simulink model "joint_test"  (R2022a)
settings: Solver=FixedStepAuto  StartTime=0.0  StopTime=2  FixedStep=0.001  RelTol=1e-3
undefined symbols (not defined in the file or in its folder): duration, effort, fins_rev1, index, joint_name, model_missile, model_name
libraries: robotlib x21, simulink_extras x8, robotgazebolib x5, simulink x1
settings Model: Creator=abiyyumufti  LastModifiedBy=abiyyumufti

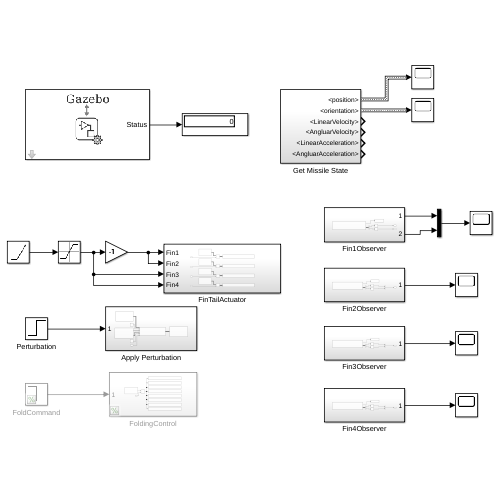
[thumbnail: Simulink's stored preview of the top-level diagram]
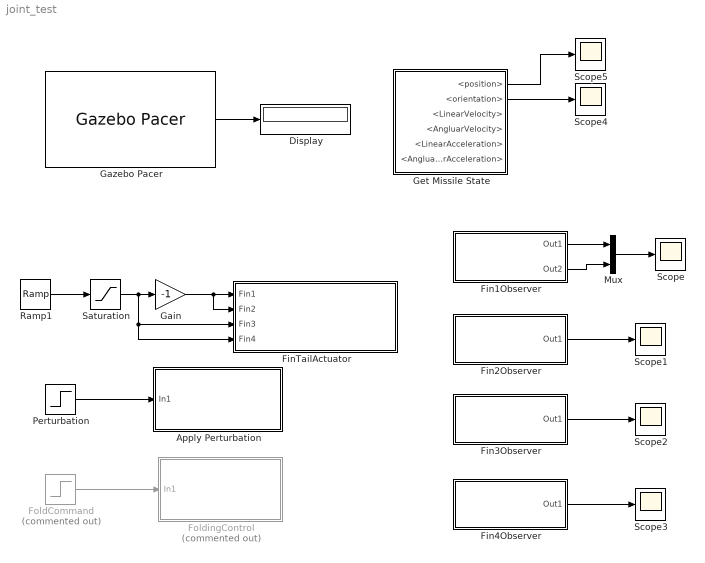
== system joint_test ==
  Apply Perturbation : Subsystem
  Display : Display
  Fin1Observer : Subsystem
  Fin2Observer : Subsystem
  Fin3Observer : Subsystem
  Fin4Observer : Subsystem
  FinTailActuator : Subsystem
  FoldCommand : Step  Commented=on  Time=0.5  Before=deg2rad(123)  After=0  SampleTime=0
  FoldingControl : Subsystem  Commented=on
  Gain : Gain  Gain=-1
  Gazebo Pacer : robotgazebolib/Gazebo Pacer  ResetBehavior=Reset Gazebo simulation time and scene  SampleTime=0.001
      settings: SourceProductBaseCode=RO
  Get Missile State : Subsystem
  Mux : Mux  Inputs=2
  Perturbation : Step  Time=0.25  After=2000  SampleTime=0.001
  Ramp1 : simulink/Sources/Ramp  slope=deg2rad(20)/1  start=0.5  InitialOutput=0
  Saturation : Saturate  UpperLimit=deg2rad(20)  LowerLimit=-deg2rad(20)
  Scope{,1..5} (6 alike) : Scope
  wires:
  Gazebo Pacer/1 -> Display/1
  Perturbation/1 -> Apply Perturbation/1(In1)
  Gain/1 -> FinTailActuator/2(Fin2), FinTailActuator/1(Fin1)
  Saturation/1 -> FinTailActuator/4(Fin4), FinTailActuator/3(Fin3), Gain/1
  Fin4Observer/1(Out1) -> Scope3/1
  Fin3Observer/1(Out1) -> Scope2/1
  Fin2Observer/1(Out1) -> Scope1/1
  Ramp1/1 -> Saturation/1
  FoldCommand/1 -> FoldingControl/1(In1)
  Get Missile State/2(<orientation>) -> Scope4/1
  Get Missile State/1(<position>) -> Scope5/1
  Fin1Observer/1(Out1) -> Mux/1
  Fin1Observer/2(Out2) -> Mux/2
  Mux/1 -> Scope/1

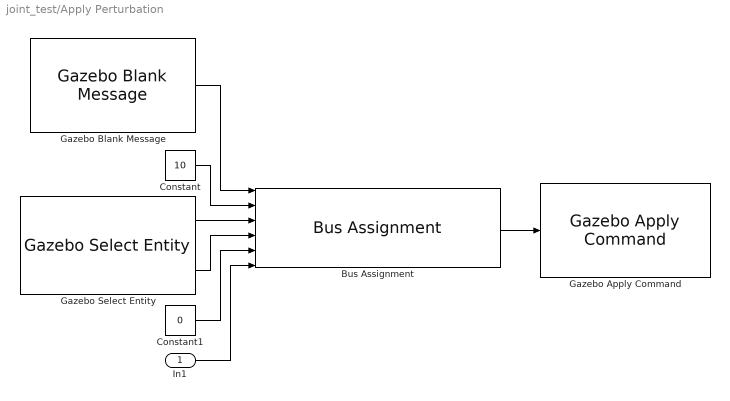
== system joint_test/Apply Perturbation ==
  In1 : Inport
  Bus Assignment : BusAssignment  AssignedSignals=duration.seconds,model_name,joint_name,index,effort
  Constant : Constant  Value=10
  Constant1 : Constant  Value=0  OutDataTypeStr=uint32
  Gazebo Apply Command : robotgazebolib/Gazebo Apply Command  cmdType=ApplyJointTorque  sampleTime=0.001
      settings: SourceProductBaseCode=RO
  Gazebo Blank Message : robotgazebolib/Gazebo Blank Message  msgType=ApplyJointTorque  sampleTime=0.001  busName='Gazebo_SL_Bus_gazebo_msgs_ApplyJointTorque'
      settings: SourceProductBaseCode=RO
  Gazebo Select Entity : robotgazebolib/Gazebo Select Entity  modelElemName=model_missile/fins_rev1  outputArraySize=128  OutputLabel=Joint  SelectType=Joint
      settings: SourceProductBaseCode=RO
  wires:
  Gazebo Select Entity/1 -> Bus Assignment/3
  Constant1/1 -> Bus Assignment/5
  In1/1 -> Bus Assignment/6
  Gazebo Select Entity/2 -> Bus Assignment/4
  Gazebo Blank Message/1 -> Bus Assignment/1
  Bus Assignment/1 -> Gazebo Apply Command/1
  Constant/1 -> Bus Assignment/2

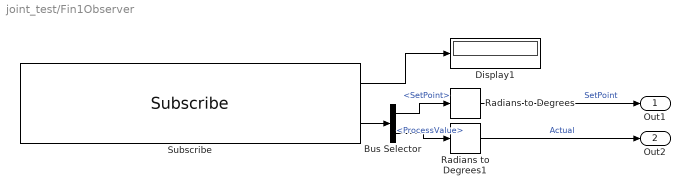
== system joint_test/Fin1Observer ==
  Bus Selector : BusSelector  OutputSignals=SetPoint,ProcessValue
  Display1 : Display
  Radians to Degrees : simulink_extras/Transformations/Radians to Degrees
  Radians to Degrees1 : simulink_extras/Transformations/Radians to Degrees
  Subscribe : robotlib/Subscribe  topicSource=Select from ROS network  topic=/model_missile_controller/fins_rev1_position_controller/state  messageType=control_msgs/JointControllerState  SampleTime=-1  legacyBusStruct=off  messageQueueLength=1
  Out1 : Outport
  Out2 : Outport  Port=2
  wires:
  Subscribe/2 -> Bus Selector/1
  Bus Selector/2 -> Radians to Degrees1/1  "<ProcessValue>"
  Subscribe/1 -> Display1/1
  Bus Selector/1 -> Radians to Degrees/1  "<SetPoint>"
  Radians to Degrees1/1 -> Out2/1  "Actual"
  Radians to Degrees/1 -> Out1/1  "SetPoint"

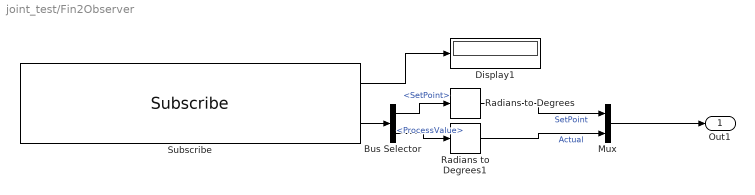
== system joint_test/Fin2Observer ==
  Bus Selector : BusSelector  OutputSignals=SetPoint,ProcessValue
  Display1 : Display
  Mux : Mux  Inputs=2
  Radians to Degrees : simulink_extras/Transformations/Radians to Degrees
  Radians to Degrees1 : simulink_extras/Transformations/Radians to Degrees
  Subscribe : robotlib/Subscribe  topicSource=Select from ROS network  topic=/model_missile_controller/fins_rev2_position_controller/state  messageType=control_msgs/JointControllerState  SampleTime=-1  legacyBusStruct=off  messageQueueLength=1
  Out1 : Outport
  wires:
  Radians to Degrees/1 -> Mux/1  "SetPoint"
  Mux/1 -> Out1/1
  Radians to Degrees1/1 -> Mux/2  "Actual"
  Bus Selector/1 -> Radians to Degrees/1  "<SetPoint>"
  Subscribe/1 -> Display1/1
  Bus Selector/2 -> Radians to Degrees1/1  "<ProcessValue>"
  Subscribe/2 -> Bus Selector/1

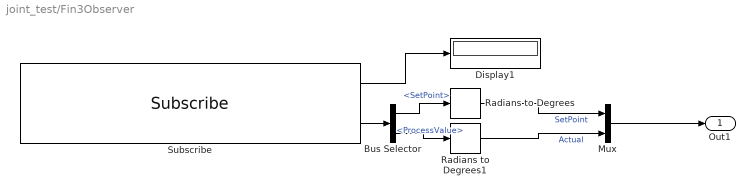
== system joint_test/Fin3Observer ==
  Bus Selector : BusSelector  OutputSignals=SetPoint,ProcessValue
  Display1 : Display
  Mux : Mux  Inputs=2
  Radians to Degrees : simulink_extras/Transformations/Radians to Degrees
  Radians to Degrees1 : simulink_extras/Transformations/Radians to Degrees
  Subscribe : robotlib/Subscribe  topicSource=Select from ROS network  topic=/model_missile_controller/fins_rev3_position_controller/state  messageType=control_msgs/JointControllerState  SampleTime=-1  legacyBusStruct=off  messageQueueLength=1
  Out1 : Outport
  wires:
  Radians to Degrees/1 -> Mux/1  "SetPoint"
  Mux/1 -> Out1/1
  Radians to Degrees1/1 -> Mux/2  "Actual"
  Bus Selector/1 -> Radians to Degrees/1  "<SetPoint>"
  Subscribe/1 -> Display1/1
  Bus Selector/2 -> Radians to Degrees1/1  "<ProcessValue>"
  Subscribe/2 -> Bus Selector/1

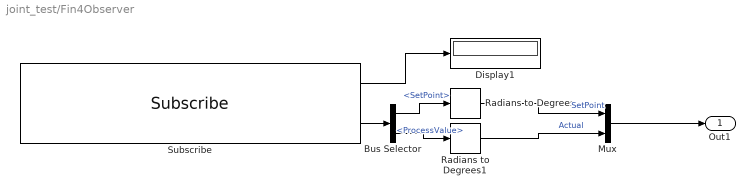
== system joint_test/Fin4Observer ==
  Bus Selector : BusSelector  OutputSignals=SetPoint,ProcessValue
  Display1 : Display
  Mux : Mux  Inputs=2
  Radians to Degrees : simulink_extras/Transformations/Radians to Degrees
  Radians to Degrees1 : simulink_extras/Transformations/Radians to Degrees
  Subscribe : robotlib/Subscribe  topicSource=Select from ROS network  topic=/model_missile_controller/fins_rev4_position_controller/state  messageType=control_msgs/JointControllerState  SampleTime=-1  legacyBusStruct=off  messageQueueLength=1
  Out1 : Outport
  wires:
  Subscribe/2 -> Bus Selector/1
  Bus Selector/2 -> Radians to Degrees1/1  "<ProcessValue>"
  Subscribe/1 -> Display1/1
  Bus Selector/1 -> Radians to Degrees/1  "<SetPoint>"
  Radians to Degrees1/1 -> Mux/2  "Actual"
  Mux/1 -> Out1/1
  Radians to Degrees/1 -> Mux/1  "SetPoint"

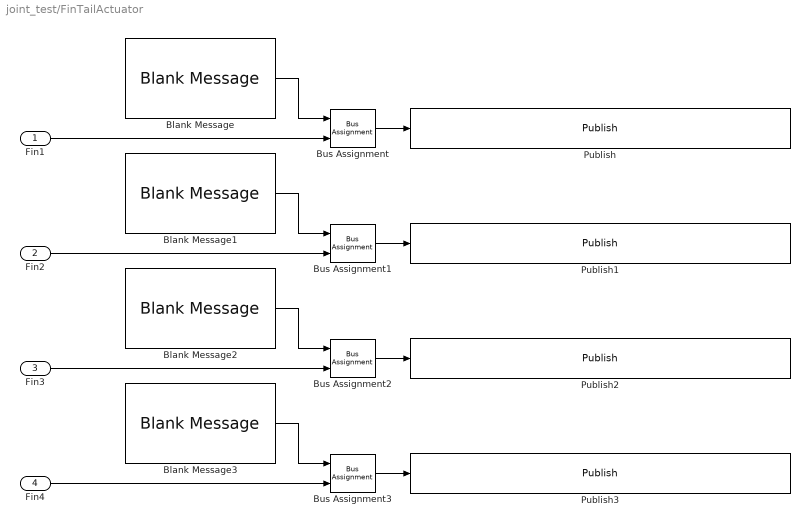
== system joint_test/FinTailActuator ==
  Fin1 : Inport
  Fin2 : Inport  Port=2
  Fin3 : Inport  Port=3
  Fin4 : Inport  Port=4
  Blank Message{,1..3} (4 alike) : robotlib/Blank Message  messageClass=Message  entityType=std_msgs/Float64  messageType=std_msgs/Float64  SampleTime=inf  legacyBusStruct=off
  Bus Assignment{,1..3} (4 alike) : BusAssignment  AssignedSignals=Data
  Publish : robotlib/Publish  topicSource=Select from ROS network  topic=/model_missile_controller/fins_rev1_position_controller/command  messageType=std_msgs/Float64  legacyBusStruct=off  messageQueueLength=1
  Publish1 : robotlib/Publish  topicSource=Select from ROS network  topic=/model_missile_controller/fins_rev2_position_controller/command  messageType=std_msgs/Float64  legacyBusStruct=off  messageQueueLength=1
  Publish2 : robotlib/Publish  topicSource=Select from ROS network  topic=/model_missile_controller/fins_rev3_position_controller/command  messageType=std_msgs/Float64  legacyBusStruct=off  messageQueueLength=1
  Publish3 : robotlib/Publish  topicSource=Select from ROS network  topic=/model_missile_controller/fins_rev4_position_controller/command  messageType=std_msgs/Float64  legacyBusStruct=off  messageQueueLength=1
  wires:
  Fin1/1 -> Bus Assignment/2
  Bus Assignment3/1 -> Publish3/1
  Blank Message/1 -> Bus Assignment/1
  Fin4/1 -> Bus Assignment3/2
  Bus Assignment1/1 -> Publish1/1
  Blank Message3/1 -> Bus Assignment3/1
  Blank Message2/1 -> Bus Assignment2/1
  Bus Assignment/1 -> Publish/1
  Blank Message1/1 -> Bus Assignment1/1
  Bus Assignment2/1 -> Publish2/1
  Fin2/1 -> Bus Assignment1/2
  Fin3/1 -> Bus Assignment2/2

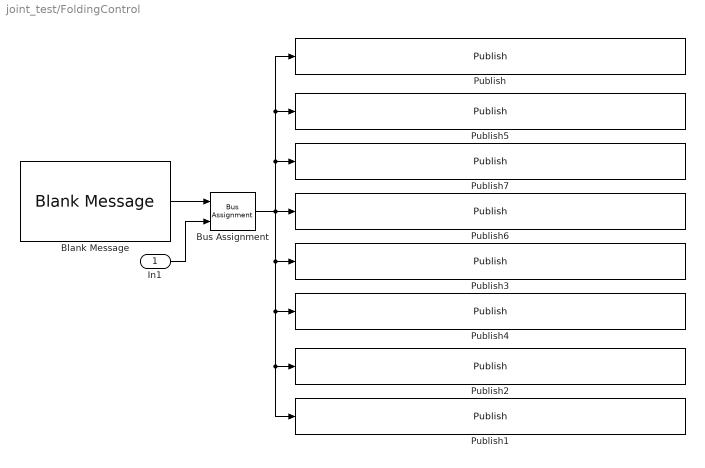
== system joint_test/FoldingControl ==
  In1 : Inport
  Blank Message : robotlib/Blank Message  messageClass=Message  entityType=std_msgs/Float64  messageType=std_msgs/Float64  SampleTime=inf  legacyBusStruct=off
  Bus Assignment : BusAssignment  AssignedSignals=Data
  Publish : robotlib/Publish  topicSource=Select from ROS network  topic=/model_missile_controller/fin_fold1_position_controller/command  messageType=std_msgs/Float64  legacyBusStruct=off  messageQueueLength=1
  Publish1 : robotlib/Publish  topicSource=Select from ROS network  topic=/model_missile_controller/fin_fold2_position_controller/command  messageType=std_msgs/Float64  legacyBusStruct=off  messageQueueLength=1
  Publish2 : robotlib/Publish  topicSource=Select from ROS network  topic=/model_missile_controller/fin_fold3_position_controller/command  messageType=std_msgs/Float64  legacyBusStruct=off  messageQueueLength=1
  Publish3 : robotlib/Publish  topicSource=Select from ROS network  topic=/model_missile_controller/fin_fold4_position_controller/command  messageType=std_msgs/Float64  legacyBusStruct=off  messageQueueLength=1
  Publish4 : robotlib/Publish  topicSource=Select from ROS network  topic=/model_missile_controller/wings_fold1_position_controller/command  messageType=std_msgs/Float64  legacyBusStruct=off  messageQueueLength=1
  Publish5 : robotlib/Publish  topicSource=Select from ROS network  topic=/model_missile_controller/wings_fold2_position_controller/command  messageType=std_msgs/Float64  legacyBusStruct=off  messageQueueLength=1
  Publish6 : robotlib/Publish  topicSource=Select from ROS network  topic=/model_missile_controller/wings_fold3_position_controller/command  messageType=std_msgs/Float64  legacyBusStruct=off  messageQueueLength=1
  Publish7 : robotlib/Publish  topicSource=Select from ROS network  topic=/model_missile_controller/wings_fold4_position_controller/command  messageType=std_msgs/Float64  legacyBusStruct=off  messageQueueLength=1
  wires:
  Bus Assignment/1 -> Publish1/1, Publish2/1, Publish4/1, Publish3/1, Publish5/1, Publish/1, Publish7/1, Publish6/1
  Blank Message/1 -> Bus Assignment/1
  In1/1 -> Bus Assignment/2

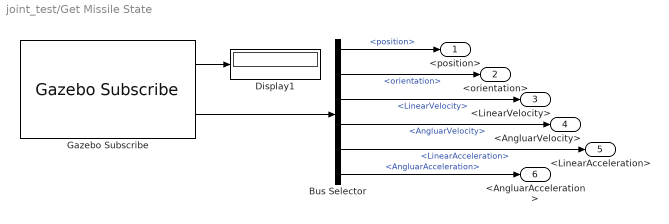
== system joint_test/Get Missile State ==
  Bus Selector : BusSelector  OutputSignals=Pose.position,Pose.orientation,LinearVelocity,AngluarVelocity,LinearAcceleration,AngluarAcceleration
  Display1 : Display
  Gazebo Subscribe : robotgazebolib/Gazebo Subscribe  topicSource=From Gazebo  topic=/gazebo/my_world/DynamicState  messageType=gazebo_msgs/custom/ssm_msgs_msgs/DynamicState  sampleTime=0.001
      settings: SourceProductBaseCode=RO
  <position> : Outport
  <orientation> : Outport  Port=2
  <LinearVelocity> : Outport  Port=3
  <AngluarVelocity> : Outport  Port=4
  <LinearAcceleration> : Outport  Port=5
  <AngluarAcceleration> : Outport  Port=6
  wires:
  Gazebo Subscribe/2 -> Bus Selector/1
  Gazebo Subscribe/1 -> Display1/1
  Bus Selector/4 -> <AngluarVelocity>/1  "<AngluarVelocity>"
  Bus Selector/6 -> <AngluarAcceleration>/1  "<AngluarAcceleration>"
  Bus Selector/5 -> <LinearAcceleration>/1  "<LinearAcceleration>"
  Bus Selector/1 -> <position>/1  "<position>"
  Bus Selector/3 -> <LinearVelocity>/1  "<LinearVelocity>"
  Bus Selector/2 -> <orientation>/1  "<orientation>"
